simulink subsystem "StudentTemplate_M2_Copy"  (R2025a)
settings: Solver=VariableStepAuto  StartTime=0.0  StopTime=10.0  RelTol=1e-3
libraries: slpidlib x7, simulink x5, eeGeneralControl x3, dspstat3 x3, cstblocks x1
(part 2 of 2)

== stateflow chart StudentTemplate_M2_Copy/draft2_Maze_exploration1 ==
  settings: updateMethod=CONTINUOUS  sampleTime=0.005
  state Left_turn1
    entry:
    theta = Z_theta;
    turn_indicator = 1;
    Z_angle = Z_angle +pi/2;
    during:
    LW = -1;
    RW = 1;
  state Go_straight
    during:
    LW = 1;
    RW = 1;
  state left_turn_setup
    entry:
    start_dist = dist_trav;
    end_dist = start_dist + 0.14;
    turn_indicator = 1;
  state Go_straight1
    entry:
    turn_indicator = 0;
    during:
    LW = 1;
    RW = 1;
  state set_Z_angle
    entry:
    Z_angle = 0;
  state Start
    entry:
    LW = 0;
    RW =0;
    turn_indicator = 0;
  state Full_rotation
    entry:
    theta = Z_theta;
    Z_angle = Z_angle - pi;
    turn_indicator = 1;
    during:
    LW = 1;
    RW =-1;
  state Left_turn
    entry:
    theta = Z_theta;
    turn_indicator = 1;
    Z_angle = Z_angle + pi/2;
    during:
    LW = -1;
    RW = 1;
  state Left_turn2
    entry:
    theta = Z_theta;
    turn_indicator = 1;
    Z_angle = Z_angle +pi/2;
    during:
    LW = -1;
    RW = 1;
  state left_turn_setup1
    entry:
    start_dist = dist_trav;
    end_dist = start_dist + 0.14;
    turn_indicator = 1;
  state right_turn
    entry:
    theta =Z_theta;
    turn_indicator = 1;
    Z_angle = Z_angle - pi/2;
    during:
    LW = 1;
    RW =-1;
  left_turn_setup -> Left_turn1 [order 2] : [dist_trav >= end_dist  ]
  Go_straight -> left_turn_setup [order 2] : [TOF_F ==0 && TOF_L ==0]
  Start -> Go_straight [order 4] : [TOF_L == 1 && TOF_F == 0 || TOF_R == 1 && TOF_F ==0]
  Go_straight -> (junction 107) [order 1] : [TOF_F ==1  ]
  Left_turn1 -> Go_straight1 : [Z_theta >= theta + pi/2]
  left_turn_setup -> (junction 103) [order 1] : [TOF_L ==1 ]
  (default) -> set_Z_angle
  (junction 103) -> (junction 107)
  Go_straight1 -> (junction 103) [order 1] : [TOF_F ==1  ]
  left_turn_setup1 -> (junction 103) [order 1] : [TOF_L ==1 ]
  (junction 107) -> Start
  Full_rotation -> (junction 103) : [Z_theta <= theta - pi && TOF_F == 0 ]
  set_Z_angle -> Start
  Go_straight1 -> left_turn_setup1 [order 2] : [TOF_F ==0 && TOF_L ==0]
  Start -> Full_rotation [order 1] : [TOF_L == 1 && TOF_R == 1 && TOF_F ==1]
  Start -> Left_turn [order 2] : [TOF_L ==0 && TOF_F ==1]
  Left_turn2 -> Start : [Z_theta >= theta + pi/2]
  Left_turn -> Start : [Z_theta>= theta +pi/2]
  right_turn -> Start : [Z_theta <= theta - pi/2]
  Start -> right_turn [order 3] : [TOF_R ==0 && TOF_F ==1]
  left_turn_setup1 -> Left_turn2 [order 2] : [dist_trav >= end_dist  ]
  data: TOF_L input; TOF_R input; LW output; RW output; dist_trav input; start_dist local; TOF_F input; end_dist local; Z_theta input; turn_indicator output; theta local; Z_angle output

== stateflow chart StudentTemplate_M2_Copy/DIstance measurement /convert_encoder_signal_to_ticks3/Chart ==
  state default
    during:
    count =0;
  state encoder_pulse_start
    during:
  state encoder_pulse_end
    during:
    count = 1;
  (default) -> default
  default -> encoder_pulse_start : [rising_edge == 1]
  encoder_pulse_start -> encoder_pulse_end : [falling_edge == 1]
  data: rising_edge input; count output; falling_edge input

== stateflow chart StudentTemplate_M2_Copy/draft2_Maze_exploration ==
  settings: updateMethod=CONTINUOUS  sampleTime=0.005
  state Left_turn1
    entry:
    theta = Z_theta;
    turn_indicator = 1;
    Z_angle = Z_angle +pi/2;
    during:
    LW = -1;
    RW = 1;
  state Go_straight
    during:
    LW = 1;
    RW = 1;
  state left_turn_setup
    entry:
    start_dist = dist_trav;
    end_dist = start_dist + 0.14;
    turn_indicator = 1;
  state Go_straight1
    entry:
    turn_indicator = 0;
    during:
    LW = 1;
    RW = 1;
  state set_Z_angle
    entry:
    Z_angle = 0;
  state Start
    entry:
    LW = 0;
    RW =0;
    turn_indicator = 0;
  state Full_rotation
    entry:
    theta = Z_theta;
    Z_angle = Z_angle - pi;
    turn_indicator = 1;
    during:
    LW = 1;
    RW =-1;
  state Left_turn
    entry:
    theta = Z_theta;
    turn_indicator = 1;
    Z_angle = Z_angle + pi/2;
    during:
    LW = -1;
    RW = 1;
  state Left_turn2
    entry:
    theta = Z_theta;
    turn_indicator = 1;
    Z_angle = Z_angle +pi/2;
    during:
    LW = -1;
    RW = 1;
  state left_turn_setup1
    entry:
    start_dist = dist_trav;
    end_dist = start_dist + 0.14;
    turn_indicator = 1;
  state right_turn
    entry:
    theta =Z_theta;
    turn_indicator = 1;
    Z_angle = Z_angle - pi/2;
    during:
    LW = 1;
    RW =-1;
  left_turn_setup -> Left_turn1 [order 2] : [dist_trav >= end_dist  ]
  Go_straight -> left_turn_setup [order 2] : [TOF_F ==0 && TOF_L ==0]
  Start -> Go_straight [order 4] : [TOF_L == 1 && TOF_F == 0 || TOF_R == 1 && TOF_F ==0]
  Go_straight -> (junction 107) [order 1] : [TOF_F ==1  ]
  Left_turn1 -> Go_straight1 : [Z_theta >= Z_angle]
  left_turn_setup -> (junction 103) [order 1] : [TOF_L ==1 ]
  (default) -> set_Z_angle
  (junction 103) -> (junction 107)
  Go_straight1 -> (junction 103) [order 1] : [TOF_F ==1  ]
  left_turn_setup1 -> (junction 103) [order 1] : [TOF_L ==1 ]
  (junction 107) -> Start
  Full_rotation -> (junction 103) : [Z_theta <= Z_angle && TOF_F == 0 ]
  set_Z_angle -> Start
  Go_straight1 -> left_turn_setup1 [order 2] : [TOF_F ==0 && TOF_L ==0]
  Start -> Full_rotation [order 1] : [TOF_L == 1 && TOF_R == 1 && TOF_F ==1]
  Start -> Left_turn [order 2] : [TOF_L ==0 && TOF_F ==1]
  Left_turn2 -> Start : [Z_theta >= Z_angle]
  Left_turn -> Start : [Z_theta >= Z_angle]
  right_turn -> Start : [Z_theta <= Z_angle]
  Start -> right_turn [order 3] : [TOF_R ==0 && TOF_F ==1]
  left_turn_setup1 -> Left_turn2 [order 2] : [dist_trav >= end_dist  ]
  data: TOF_L input; TOF_R input; LW output; RW output; dist_trav input; start_dist local; TOF_F input; end_dist local; Z_theta input; turn_indicator output; theta local; Z_angle output
